simulink model "Simscape"  (R2021b)
(part 17 of 40)

  pan_cross_head_am_77_RIGID : Subsystem
  pan_cross_head_am_78_RIGID : Subsystem
  pan_cross_head_am_79_RIGID : Subsystem
  pan_cross_head_am_80_RIGID : Subsystem
  pan_cross_head_am_81_RIGID : Subsystem
  pan_cross_head_am_82_RIGID : Subsystem
  pan_cross_head_am_83_RIGID : Subsystem
  pan_cross_head_am_84_RIGID : Subsystem
  pan_cross_head_am_85_RIGID : Subsystem
  pan_cross_head_am_86_RIGID : Subsystem
  pan_cross_head_am_87_RIGID : Subsystem
  pan_cross_head_am_88_RIGID : Subsystem
  pan_cross_head_am_89_RIGID : Subsystem
  pan_cross_head_am_8_RIGID : Subsystem
  pan_cross_head_am_90_RIGID : Subsystem
  pan_cross_head_am_91_RIGID : Subsystem
  socket_set_screw_cone_point_am_2_RIGID : Subsystem
  socket_set_screw_cone_point_am_3_RIGID : Subsystem
  F : PMIOPort  Side=Right
  connections:
  Transform/RConn1 -- instrument_ball_bearing_68_am_7_RIGID/LConn1
  Transform1/RConn1 -- instrument_ball_bearing_68_am_16_RIGID/LConn1
  Transform10/RConn1 -- instrument_ball_bearing_68_am_29_RIGID/LConn1
  Joint2_Ring_Spacers_62_RIGID/LConn1 -- Transform100/RConn1
  Transform101/RConn1 -- instrument_ball_bearing_68_am_126_RIGID/LConn1
  Joint2_Ring_Spacers_64_RIGID/LConn1 -- Transform102/RConn1
  Transform103/RConn1 -- instrument_ball_bearing_68_am_134_RIGID/LConn1
  Joint2_Ring_Spacers_65_RIGID/LConn1 -- Transform104/RConn1
  Joint2_Ring_Spacers_63_RIGID/LConn1 -- Transform105/RConn1
  Joint2_Ring_Spacers_66_RIGID/LConn1 -- Transform106/RConn1
  Joint2_Ring_Spacers_67_RIGID/LConn1 -- Transform107/RConn1
  Transform108/RConn1 -- instrument_ball_bearing_68_am_139_RIGID/LConn1
  Transform109/RConn1 -- instrument_ball_bearing_68_am_140_RIGID/LConn1
  Transform11/RConn1 -- formed_hex_screw_am_8_RIGID/LConn1
  Transform110/RConn1 -- instrument_ball_bearing_68_am_138_RIGID/LConn1
  Transform111/RConn1 -- instrument_ball_bearing_68_am_141_RIGID/LConn1
  Transform112/RConn1 -- instrument_ball_bearing_68_am_143_RIGID/LConn1
  Transform113/RConn1 -- instrument_ball_bearing_68_am_142_RIGID/LConn1
  Transform114/RConn1 -- instrument_ball_bearing_68_am_144_RIGID/LConn1
  Transform115/RConn1 -- instrument_ball_bearing_68_am_145_RIGID/LConn1
  Joint2_Ring_Spacers_77_RIGID/LConn1 -- Transform116/RConn1
  Transform117/RConn1 -- instrument_ball_bearing_68_am_149_RIGID/LConn1
  Joint2_Ring_Spacers_69_RIGID/LConn1 -- Transform118/RConn1
  Joint2_Ring_Spacers_72_RIGID/LConn1 -- Transform119/RConn1
  Transform12/RConn1 -- instrument_ball_bearing_68_am_17_RIGID/LConn1
  Joint2_Ring_Spacers_70_RIGID/LConn1 -- Transform120/RConn1
  Joint2_Ring_Spacers_73_RIGID/LConn1 -- Transform121/RConn1
  Joint2_Ring_Spacers_74_RIGID/LConn1 -- Transform122/RConn1
  Transform123/RConn1 -- instrument_ball_bearing_68_am_148_RIGID/LConn1
  Transform124/RConn1 -- instrument_ball_bearing_68_am_146_RIGID/LConn1
  Joint2_Ring_Spacers_71_RIGID/LConn1 -- Transform125/RConn1
  Transform126/RConn1 -- instrument_ball_bearing_68_am_147_RIGID/LConn1
  Joint2_Ring_Spacers_75_RIGID/LConn1 -- Transform127/RConn1
  Joint2_Ring_Spacers_76_RIGID/LConn1 -- Transform128/RConn1
  Joint2_Ring_Spacers_68_RIGID/LConn1 -- Transform129/RConn1
  Joint2_Output_Shaft_1_RIGID/LConn1 -- Transform13/RConn1
  Transform130/RConn1 -- instrument_ball_bearing_68_am_151_RIGID/LConn1
  Joint2_Ring_Spacers_78_RIGID/LConn1 -- Transform131/RConn1
  Joint2_Ring_Spacers_80_RIGID/LConn1 -- Transform132/RConn1
  Transform133/RConn1 -- instrument_ball_bearing_68_am_162_RIGID/LConn1
  Transform134/RConn1 -- instrument_ball_bearing_68_am_154_RIGID/LConn1
  Transform135/RConn1 -- instrument_ball_bearing_68_am_153_RIGID/LConn1
  Transform136/RConn1 -- instrument_ball_bearing_68_am_155_RIGID/LConn1
  Transform137/RConn1 -- instrument_ball_bearing_68_am_156_RIGID/LConn1
  Transform138/RConn1 -- instrument_ball_bearing_68_am_152_RIGID/LConn1
  Transform139/RConn1 -- instrument_ball_bearing_68_am_158_RIGID/LConn1
  Transform14/RConn1 -- instrument_ball_bearing_68_am_9_RIGID/LConn1
  Transform140/RConn1 -- instrument_ball_bearing_68_am_161_RIGID/LConn1
  Transform141/RConn1 -- instrument_ball_bearing_68_am_157_RIGID/LConn1
  Transform142/RConn1 -- instrument_ball_bearing_68_am_159_RIGID/LConn1
  Joint2_Ring_Spacers_79_RIGID/LConn1 -- Transform143/RConn1
  Transform144/RConn1 -- instrument_ball_bearing_68_am_160_RIGID/LConn1
  Transform145/RConn1 -- instrument_ball_bearing_68_am_150_RIGID/LConn1
  Transform146/RConn1 -- pan_cross_head_am_82_RIGID/LConn1
  Transform147/RConn1 -- pan_cross_head_am_85_RIGID/LConn1
  Transform148/RConn1 -- pan_cross_head_am_86_RIGID/LConn1
  Transform149/RConn1 -- pan_cross_head_am_79_RIGID/LConn1
  Transform15/RConn1 -- instrument_ball_bearing_68_am_12_RIGID/LConn1
  Transform150/RConn1 -- pan_cross_head_am_80_RIGID/LConn1
  Transform151/RConn1 -- pan_cross_head_am_81_RIGID/LConn1
  Transform152/RConn1 -- pan_cross_head_am_83_RIGID/LConn1
  Transform153/RConn1 -- pan_cross_head_am_84_RIGID/LConn1
  Transform154/RConn1 -- pan_cross_head_am_89_RIGID/LConn1
  Transform155/RConn1 -- pan_cross_head_am_90_RIGID/LConn1
  Transform156/RConn1 -- pan_cross_head_am_88_RIGID/LConn1
  Transform157/RConn1 -- pan_cross_head_am_87_RIGID/LConn1
  Transform158/RConn1 -- formed_hex_screw_am_19_RIGID/LConn1
  Transform159/RConn1 -- pan_cross_head_am_91_RIGID/LConn1
  Transform16/RConn1 -- instrument_ball_bearing_68_am_14_RIGID/LConn1
  Transform160/RConn1 -- pan_cross_head_am_78_RIGID/LConn1
  Transform/LConn1 -- ReferenceFrame/RConn1 -- Transform1/LConn1 -- Transform10/LConn1 -- Transform100/LConn1 -- Transform101/LConn1 -- Transform102/LConn1 -- Transform103/LConn1 -- Transform104/LConn1 -- Transform105/LConn1 -- Transform106/LConn1 -- Transform107/LConn1 -- Transform108/LConn1 -- Transform109/LConn1 -- Transform11/LConn1 -- Transform110/LConn1 -- Transform111/LConn1 -- Transform112/LConn1 -- Transform113/LConn1 -- Transform114/LConn1 -- Transform115/LConn1 -- Transform116/LConn1 -- Transform117/LConn1 -- Transform118/LConn1 -- Transform119/LConn1 -- Transform12/LConn1 -- Transform120/LConn1 -- Transform121/LConn1 -- Transform122/LConn1 -- Transform123/LConn1 -- Transform124/LConn1 -- Transform125/LConn1 -- Transform126/LConn1 -- Transform127/LConn1 -- Transform128/LConn1 -- Transform129/LConn1 -- Transform13/LConn1 -- Transform130/LConn1 -- Transform131/LConn1 -- Transform132/LConn1 -- Transform133/LConn1 -- Transform134/LConn1 -- Transform135/LConn1 -- Transform136/LConn1 -- Transform137/LConn1 -- Transform138/LConn1 -- Transform139/LConn1 -- Transform14/LConn1 -- Transform140/LConn1 -- Transform141/LConn1 -- Transform142/LConn1 -- Transform143/LConn1 -- Transform144/LConn1 -- Transform145/LConn1 -- Transform146/LConn1 -- Transform147/LConn1 -- Transform148/LConn1 -- Transform149/LConn1 -- Transform15/LConn1 -- Transform150/LConn1 -- Transform151/LConn1 -- Transform152/LConn1 -- Transform153/LConn1 -- Transform154/LConn1 -- Transform155/LConn1 -- Transform156/LConn1 -- Transform157/LConn1 -- Transform158/LConn1 -- Transform159/LConn1 -- Transform16/LConn1 -- Transform160/LConn1 -- Transform161/RConn1 -- Transform17/LConn1 -- Transform18/LConn1 -- Transform19/LConn1 -- Transform2/LConn1 -- Transform20/LConn1 -- Transform21/LConn1 -- Transform22/LConn1 -- Transform23/LConn1 -- Transform24/LConn1 -- Transform25/LConn1 -- Transform26/LConn1 -- Transform27/LConn1 -- Transform28/LConn1 -- Transform29/LConn1 -- Transform3/LConn1 -- Transform30/LConn1 -- Transform31/LConn1 -- Transform32/LConn1 -- Transform33/LConn1 -- Transform34/LConn1 -- Transform35/LConn1 -- Transform36/LConn1 -- Transform37/LConn1 -- Transform38/LConn1 -- Transform39/LConn1 -- Transform4/LConn1 -- Transform40/LConn1 -- Transform41/LConn1 -- Transform42/LConn1 -- Transform43/LConn1 -- Transform44/LConn1 -- Transform45/LConn1 -- Transform46/LConn1 -- Transform47/LConn1 -- Transform48/LConn1 -- Transform49/LConn1 -- Transform5/LConn1 -- Transform50/LConn1 -- Transform51/LConn1 -- Transform52/LConn1 -- Transform53/LConn1 -- Transform54/LConn1 -- Transform55/LConn1 -- Transform56/LConn1 -- Transform57/LConn1 -- Transform58/LConn1 -- Transform59/LConn1 -- Transform6/LConn1 -- Transform60/LConn1 -- Transform61/LConn1 -- Transform62/LConn1 -- Transform63/LConn1 -- Transform64/LConn1 -- Transform65/LConn1 -- Transform66/LConn1 -- Transform67/LConn1 -- Transform68/LConn1 -- Transform69/LConn1 -- Transform7/LConn1 -- Transform70/LConn1 -- Transform71/LConn1 -- Transform72/LConn1 -- Transform73/LConn1 -- Transform74/LConn1 -- Transform75/LConn1 -- Transform76/LConn1 -- Transform77/LConn1 -- Transform78/LConn1 -- Transform79/LConn1 -- Transform8/LConn1 -- Transform80/LConn1 -- Transform81/LConn1 -- Transform82/LConn1 -- Transform83/LConn1 -- Transform84/LConn1 -- Transform85/LConn1 -- Transform86/LConn1 -- Transform87/LConn1 -- Transform88/LConn1 -- Transform89/LConn1 -- Transform9/LConn1 -- Transform90/LConn1 -- Transform91/LConn1 -- Transform92/LConn1 -- Transform93/LConn1 -- Transform94/LConn1 -- Transform95/LConn1 -- Transform96/LConn1 -- Transform97/LConn1 -- Transform98/LConn1 -- Transform99/LConn1
  Transform161/LConn1 -- F/RConn1
  Transform17/RConn1 -- formed_hex_screw_am_7_RIGID/LConn1
  Joint2_Cyclo_Disk_Version2_1_RIGID/LConn1 -- Transform18/RConn1
  Transform19/RConn1 -- instrument_ball_bearing_68_am_18_RIGID/LConn1
  Transform2/RConn1 -- instrument_ball_bearing_68_am_10_RIGID/LConn1
  Transform20/RConn1 -- instrument_ball_bearing_68_am_21_RIGID/LConn1
  Transform21/RConn1 -- instrument_ball_bearing_68_am_20_RIGID/LConn1
  Transform22/RConn1 -- instrument_ball_bearing_68_am_23_RIGID/LConn1
  Transform23/RConn1 -- formed_hex_screw_am_9_RIGID/LConn1
  Transform24/RConn1 -- instrument_ball_bearing_68_am_19_RIGID/LConn1
  Transform25/RConn1 -- instrument_ball_bearing_68_am_25_RIGID/LConn1
  Transform26/RConn1 -- instrument_ball_bearing_68_am_24_RIGID/LConn1
  Transform27/RConn1 -- instrument_ball_bearing_68_am_26_RIGID/LConn1
  Transform28/RConn1 -- instrument_ball_bearing_68_am_27_RIGID/LConn1
  Transform29/RConn1 -- instrument_ball_bearing_68_am_22_RIGID/LConn1
  Joint2_Cyclo_Disk_Version2_3_RIGID/LConn1 -- Transform3/RConn1
  Transform30/RConn1 -- formed_hex_screw_am_11_RIGID/LConn1
  Transform31/RConn1 -- formed_hex_screw_am_12_RIGID/LConn1
  Transform32/RConn1 -- instrument_ball_bearing_68_am_44_RIGID/LConn1
  Transform33/RConn1 -- instrument_ball_bearing_68_am_33_RIGID/LConn1
  Transform34/RConn1 -- hex_nut_style_2_ams_4_RIGID/LConn1
  Transform35/RConn1 -- instrument_ball_bearing_68_am_35_RIGID/LConn1
  Transform36/RConn1 -- instrument_ball_bearing_68_am_80_RIGID/LConn1
  Transform37/RConn1 -- pan_cross_head_am_75_RIGID/LConn1
  Transform38/RConn1 -- instrument_ball_bearing_68_am_30_RIGID/LConn1
  Transform39/RConn1 -- instrument_ball_bearing_68_am_32_RIGID/LConn1
  Transform4/RConn1 -- socket_set_screw_cone_point_am_2_RIGID/LConn1
  Joint2_Ring_Spacers_5_RIGID/LConn1 -- Transform40/RConn1
  Transform41/RConn1 -- instrument_ball_bearing_68_am_45_RIGID/LConn1
  Transform42/RConn1 -- pan_cross_head_am_73_RIGID/LConn1
  Transform43/RConn1 -- formed_hex_screw_am_13_RIGID/LConn1
  Transform44/RConn1 -- instrument_ball_bearing_68_am_38_RIGID/LConn1
  Joint2_Ring_Spacers_6_RIGID/LConn1 -- Transform45/RConn1
  Transform46/RConn1 -- instrument_ball_bearing_68_am_43_RIGID/LConn1
  Transform47/RConn1 -- pan_cross_head_am_8_RIGID/LConn1
  Transform48/RConn1 -- instrument_ball_bearing_68_am_37_RIGID/LConn1
  Transform49/RConn1 -- pan_cross_head_am_74_RIGID/LConn1
  Transform5/RConn1 -- instrument_ball_bearing_68_am_13_RIGID/LConn1
  Transform50/RConn1 -- instrument_ball_bearing_68_am_34_RIGID/LConn1
  Transform51/RConn1 -- socket_set_screw_cone_point_am_3_RIGID/LConn1
  Transform52/RConn1 -- instrument_ball_bearing_68_am_81_RIGID/LConn1
  Joint2_Top_Case_1_RIGID/LConn1 -- Transform53/RConn1
  Transform54/RConn1 -- instrument_ball_bearing_68_am_83_RIGID/LConn1
  Transform55/RConn1 -- instrument_ball_bearing_68_am_31_RIGID/LConn1
  Transform56/RConn1 -- instrument_ball_bearing_68_am_84_RIGID/LConn1
  Transform57/RConn1 -- pan_cross_head_am_76_RIGID/LConn1
  Transform58/RConn1 -- pan_cross_head_am_77_RIGID/LConn1
  Transform59/RConn1 -- formed_hex_screw_am_5_RIGID/LConn1
  Transform6/RConn1 -- formed_hex_screw_am_10_RIGID/LConn1
  Joint2_Cover_1_RIGID/LConn1 -- Transform60/RConn1
  Transform61/RConn1 -- formed_hex_screw_am_2_RIGID/LConn1
  Transform62/RConn1 -- formed_hex_screw_am_6_RIGID/LConn1
  Joint_2_main_case_2_RIGID/LConn1 -- Transform63/RConn1
  NEMA23_Cyclo_1_RIGID/LConn1 -- Transform64/RConn1
  Transform65/RConn1 -- formed_hex_screw_am_4_RIGID/LConn1
  Transform66/RConn1 -- hex_nut_style_2_ams_2_RIGID/LConn1
  Joint2_Eccentric_Shaft_Version2_1_RIGID/LConn1 -- Transform67/RConn1
  Transform68/RConn1 -- pan_cross_head_am_61_RIGID/LConn1
  Transform69/RConn1 -- pan_cross_head_am_66_RIGID/LConn1
  Transform7/RConn1 -- instrument_ball_bearing_68_am_15_RIGID/LConn1
  Transform70/RConn1 -- pan_cross_head_am_60_RIGID/LConn1
  Transform71/RConn1 -- pan_cross_head_am_65_RIGID/LConn1
  Transform72/RConn1 -- pan_cross_head_am_71_RIGID/LConn1
  Transform73/RConn1 -- pan_cross_head_am_59_RIGID/LConn1
  Transform74/RConn1 -- pan_cross_head_am_62_RIGID/LConn1
  Transform75/RConn1 -- pan_cross_head_am_63_RIGID/LConn1
  Transform76/RConn1 -- pan_cross_head_am_64_RIGID/LConn1
  Transform77/RConn1 -- pan_cross_head_am_67_RIGID/LConn1
  Transform78/RConn1 -- pan_cross_head_am_68_RIGID/LConn1
  Transform79/RConn1 -- pan_cross_head_am_69_RIGID/LConn1
  Transform8/RConn1 -- instrument_ball_bearing_68_am_28_RIGID/LConn1
  Transform80/RConn1 -- pan_cross_head_am_70_RIGID/LConn1
  Transform81/RConn1 -- instrument_ball_bearing_68_am_133_RIGID/LConn1
  Transform82/RConn1 -- instrument_ball_bearing_68_am_136_RIGID/LConn1
  Joint2_Ring_Spacers_55_RIGID/LConn1 -- Transform83/RConn1
  Joint2_Ring_Spacers_59_RIGID/LConn1 -- Transform84/RConn1
  Joint2_Ring_Spacers_58_RIGID/LConn1 -- Transform85/RConn1
  Transform86/RConn1 -- instrument_ball_bearing_68_am_137_RIGID/LConn1
  Transform87/RConn1 -- instrument_ball_bearing_68_am_130_RIGID/LConn1
  Transform88/RConn1 -- instrument_ball_bearing_68_am_125_RIGID/LConn1
  Transform89/RConn1 -- instrument_ball_bearing_68_am_135_RIGID/LConn1
  Transform9/RConn1 -- instrument_ball_bearing_68_am_8_RIGID/LConn1
  Joint2_Ring_Spacers_56_RIGID/LConn1 -- Transform90/RConn1
  Transform91/RConn1 -- instrument_ball_bearing_68_am_128_RIGID/LConn1
  Transform92/RConn1 -- instrument_ball_bearing_68_am_131_RIGID/LConn1
  Transform93/RConn1 -- instrument_ball_bearing_68_am_127_RIGID/LConn1
  Transform94/RConn1 -- instrument_ball_bearing_68_am_124_RIGID/LConn1
  Transform95/RConn1 -- instrument_ball_bearing_68_am_132_RIGID/LConn1
  Joint2_Ring_Spacers_57_RIGID/LConn1 -- Transform96/RConn1
  Joint2_Ring_Spacers_60_RIGID/LConn1 -- Transform97/RConn1
  Joint2_Ring_Spacers_61_RIGID/LConn1 -- Transform98/RConn1
  Transform99/RConn1 -- instrument_ball_bearing_68_am_129_RIGID/LConn1
